simulink model "daolibai"  (R2021b)
settings: Solver=VariableStepAuto  StartTime=0.0  StopTime=3  MaxStep=1e-3  RelTol=1e-3
values from neighbouring files (symbols this model uses):
  A = [0 1 0 0 ... (first row only)    [v4.m]
  B = [0;1;0;4.9]    [v4.m]
  C = [1 0 0 0 ... (first row only)    [v4.m]
  K = abs(p1^2*(p1+10)*(p1+p)/(10*p1))    [v1.m]    (also in v2.m = abs((p1 + p) * (p1^2 + 0.1 * p1 + 4) * p1/((2*p1+0.1)*(p1+z); v4.m = double([k.k1,k.k2,k.k3,k.k4]))
  L = 1    [v3.m]    (also in v4.m = double([l.L1_1,l.L1_2;            l.L2_1,l.L2_2;            )
libraries: cstblocks x2
settings Model: Creator=Administrator  LastModifiedBy=Administrator

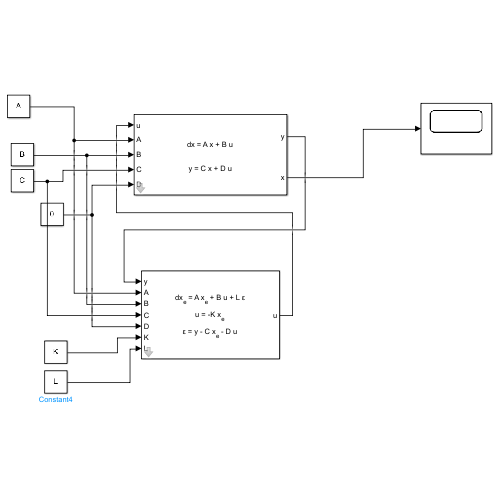
[thumbnail: Simulink's stored preview of the top-level diagram]
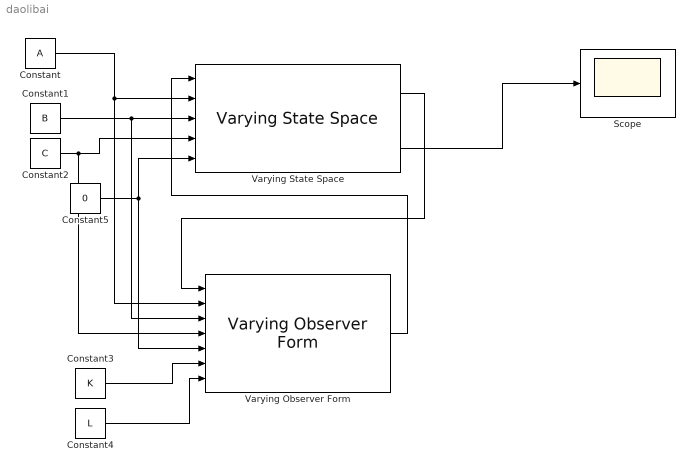
== system daolibai ==
  Constant : Constant  Value=A
  Constant1 : Constant  Value=B  VectorParams1D=off
  Constant2 : Constant  Value=C
  Constant3 : Constant  Value=K  VectorParams1D=off
  Constant4 : Constant  Value=L
  Constant5 : Constant  Value=0
  Scope : Scope
  Varying Observer Form : cstblocks/Linear Parameter Varying/Varying Observer Form  x0=x_0  xNames=''  OutputX=off  OutputDX=off
      settings: SourceProductBaseCode=CT
  Varying State Space : cstblocks/Linear Parameter Varying/Varying State Space  x0=x_0  xNames=''  OutputX=on  OutputDX=off
  wires:
  Varying State Space/1 -> Varying Observer Form/1
  Varying Observer Form/1 -> Varying State Space/1
  Constant/1 -> Varying Observer Form/2, Varying State Space/2
  Constant1/1 -> Varying Observer Form/3, Varying State Space/3
  Constant2/1 -> Varying Observer Form/4, Varying State Space/4
  Constant5/1 -> Varying State Space/5, Varying Observer Form/5
  Constant3/1 -> Varying Observer Form/6
  Constant4/1 -> Varying Observer Form/7
  Varying State Space/2 -> Scope/1
